simulink model "s1"  (R2022a)
settings: Solver=VariableStepAuto  StartTime=0.0  StopTime=50  RelTol=1e-6
settings Model: Creator=PC  LastModifiedBy=PC

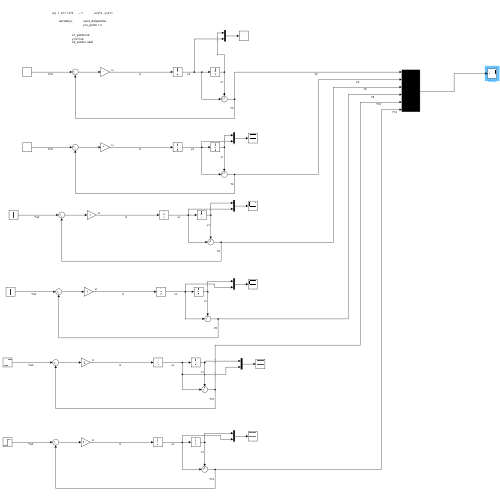
[thumbnail: Simulink's stored preview of the top-level diagram]
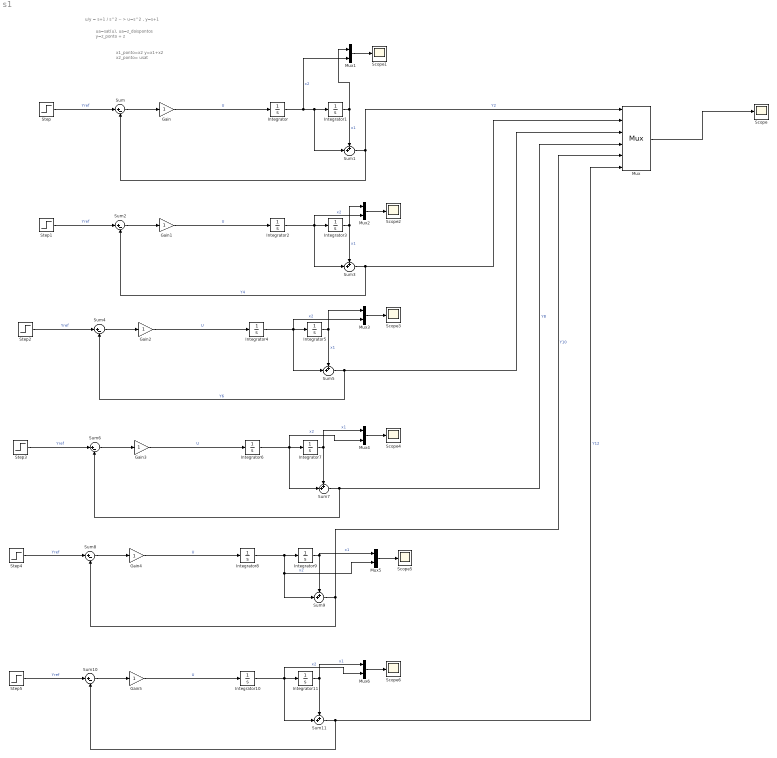
== system s1 ==
  note: x1_ponto=x2
      | y=x1+x2
      | x2_ponto= usat
  note: ua=sat(u),             ua=z_doispontos
      | 				y=z_ponto + z
  note: u/y = s+1 / s^2 -- > u=s^2 , y=s+1
  Gain{,1..5} (6 alike) : Gain
  Integrator{,1..11} (12 alike) : Integrator
  Mux : Mux  Inputs=6
  Mux{1..6} (6 alike) : Mux  Inputs=2
  Scope{,1..6} (7 alike) : Scope
  Step : Step  After=2  SampleTime=0
  Step1 : Step  After=4  SampleTime=0
  Step2 : Step  After=6  SampleTime=0
  Step3 : Step  After=8  SampleTime=0
  Step4 : Step  After=10  SampleTime=0
  Step5 : Step  After=12  SampleTime=0
  Sum{,2,4,6,8,10} (6 alike) : Sum  Inputs=|+-
  Sum{1,3,5,7,9,11} (6 alike) : Sum  Inputs=++|
  wires:
  Step/1 -> Sum/1  "Yref"
  Sum/1 -> Gain/1
  Gain/1 -> Integrator/1  "U"
  Integrator/1 -> Mux1/2, Sum1/2, Integrator1/1  "x2"
  Integrator1/1 -> Sum1/1, Mux1/1  "x1"
  Sum1/1 -> Mux/1, Sum/2  "Y2"
  Mux/1 -> Scope/1
  Gain1/1 -> Integrator2/1  "U"
  Step1/1 -> Sum2/1  "Yref"
  Sum3/1 -> Mux/2, Sum2/2  "Y4"
  Integrator3/1 -> Mux2/1, Sum3/1  "x1"
  Integrator2/1 -> Sum3/2, Integrator3/1, Mux2/2  "x2"
  Sum2/1 -> Gain1/1
  Gain2/1 -> Integrator4/1  "U"
  Step2/1 -> Sum4/1  "Yref"
  Sum5/1 -> Mux/3, Sum4/2  "Y6"
  Integrator5/1 -> Mux3/1, Sum5/1  "x1"
  Integrator4/1 -> Sum5/2, Integrator5/1, Mux3/2  "x2"
  Sum4/1 -> Gain2/1
  Gain3/1 -> Integrator6/1  "U"
  Step3/1 -> Sum6/1  "Yref"
  Sum7/1 -> Mux/4, Sum6/2  "Y8"
  Integrator7/1 -> Mux4/1, Sum7/1  "x1"
  Integrator6/1 -> Sum7/2, Integrator7/1, Mux4/2  "x2"
  Sum6/1 -> Gain3/1
  Gain4/1 -> Integrator8/1  "U"
  Step4/1 -> Sum8/1  "Yref"
  Sum9/1 -> Mux/5, Sum8/2  "Y10"
  Integrator9/1 -> Mux5/1, Sum9/1  "x1"
  Integrator8/1 -> Sum9/2, Mux5/2, Integrator9/1  "x2"
  Sum8/1 -> Gain4/1
  Gain5/1 -> Integrator10/1  "U"
  Step5/1 -> Sum10/1  "Yref"
  Sum11/1 -> Mux/6, Sum10/2  "Y12"
  Integrator11/1 -> Mux6/1, Sum11/1  "x1"
  Integrator10/1 -> Sum11/2, Integrator11/1, Mux6/2  "x2"
  Sum10/1 -> Gain5/1
  Mux1/1 -> Scope1/1
  Mux2/1 -> Scope2/1
  Mux3/1 -> Scope3/1
  Mux4/1 -> Scope4/1
  Mux5/1 -> Scope5/1
  Mux6/1 -> Scope6/1
